simulink model "net"  (R2018b)
settings: Solver=VariableStepAuto  StartTime=0.0  StopTime=10.0  RelTol=1e-3
libraries: neural x107
(part 3 of 3)

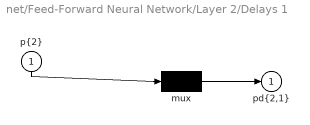
== system net/Feed-Forward Neural Network/Layer 2/Delays 1 ==
  "p{2}" : Inport  PortDimensions=100
      mask Display: e = 0.06;c1 = [120 230 180]/255;c2 = ([120 230 180]+0)/(256+128);c3 = ([120 230 180]+128)/(256+128);patch([0 1 1 0],[0 0 1 1],c1);patch([0 1 1 1-e 1-e 0+e],[0 0 1 1-e 0+e 0+e],c2);patch([0 0 1 1-e 0+e 0+e],[0 1 1 1-e 1-e 0+e],c3);plot([0 1 1 0 0],[0 0 1 1 0]);
  mux : Mux  Inputs=1
      mask Display: e = 0.06;c1 = [120 150 230]/255;c2 = ([120 150 230]+0)/383;c3 = ([120 150 230]+128)/383;patch([0 1 1 0],[0 0 1 1],c1);patch([0 1 1 1-e 1-e 0+e],[0 0 1 1-e 0+e 0+e],c2);patch([0 0 1 1-e 0+e 0+e],[0 1 1 1-e 1-e 0+e],c3);plot([0 1 1 0 0],[0 0 1 1 0]);disp('Mux')
  "pd{2,1}" : Outport
      mask Display: e = 0.06;c1 = [120 230 180]/255;c2 = ([120 230 180]+0)/(256+128);c3 = ([120 230 180]+128)/(256+128);patch([0 1 1 0],[0 0 1 1],c1);patch([0 1 1 1-e 1-e 0+e],[0 0 1 1-e 0+e 0+e],c2);patch([0 0 1 1-e 0+e 0+e],[0 1 1 1-e 1-e 0+e],c3);plot([0 1 1 0 0],[0 0 1 1 0]);
  wires:
  "p{2}"/1 -> mux/1
  mux/1 -> "pd{2,1}"/1

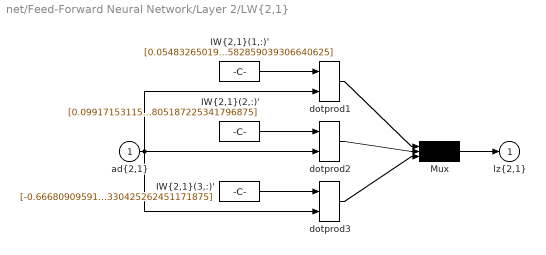
== system net/Feed-Forward Neural Network/Layer 2/LW{2,1} ==
  "ad{2,1}" : Inport  PortDimensions=100
      mask Display: e = 0.06;c1 = [120 230 180]/255;c2 = ([120 230 180]+0)/(256+128);c3 = ([120 230 180]+128)/(256+128);patch([0 1 1 0],[0 0 1 1],c1);patch([0 1 1 1-e 1-e 0+e],[0 0 1 1-e 0+e 0+e],c2);patch([0 0 1 1-e 0+e 0+e],[0 1 1 1-e 1-e 0+e],c3);plot([0 1 1 0 0],[0 0 1 1 0]);
  "IW{2,1}(1,:)'" : Constant  Value=[0.05483265019462690847973362906486727297306060791015625;0.012125815427491970499573881170363165438175201416015625;-0.1686587326797104047226838474671239964663982391357421875;-0.0202168258309454972054819421600768691860139369964599609375;0.09121870288483206745677733806587639264762401580810546875;0.353670820827776122285968085634522140026092529296875;-0.2475021717375649188408459622223745100200176239013671875;0.55673530010910587950689887293265201151371002197265625;0.015636698910315660615566457636305131018161773681640625;-0.0001195455807457557195760955437435768544673919677734375;0.3032284377369445227401456577354110777378082275390625;0.1307921379857321098061362363296211697161197662353515625;-0.244052362784950183094423437069053761661052703857421875;-0.6049096829452167423113451150129549205303192138671875;-0.3976379994996428468567728486959822475910186767578125;0.012026652977590514270733734747409471310675144195556640625;0.269113235915282855703622999499202705919742584228515625;-0.250837025003143809787076179418363608419895172119140625;0.379561693505631569944824832418817095458507537841796875;0.460939830487912372003478367332718335092067718505859375;-0.03214451578485445770727579883896396495401859283447265625;-0.0025710394266931051177049738498681108467280864715576171875;-0.52049228827995885904300621405127458274364471435546875;-0.09811246288179158170361660040725837461650371551513671875;-0.21610186479028847816863390107755549252033233642578125;0.0053971563130207067526811215429916046559810638427734375;-0.41390321109532390853047445489210076630115509033203125;-0.1428236061893602137917724803628516383469104766845703125;0.10957887134342043922163867364361067302525043487548828125;0.41999333485903267426664342565345577895641326904296875;0.11458371072683019853410968380558188073337078094482421875;0.1827573994210988372888238018276751972734928131103515625;-0.49626748851689661545805165587808005511760711669921875;-0.11629521544934078025601564831958967261016368865966796875;-0.0910286946376959449356291997901280410587787628173828125;0.323282162200989653388916167386923916637897491455078125;0.1194266060861080280819379595413920469582080841064453125;0.022955875877818811281461108819712535478174686431884765625;-0.0802221869070025850323446547918138094246387481689453125;0.000706058329053530810137662143688430660404264926910400390625;0.1055642718582814054695262484528939239680767059326171875;-0.11118762630784939648975750969839282333850860595703125;-0.288644173794616654138422973119304515421390533447265625;-0.04630920869394038186239725973791792057454586029052734375;-0.1142913256135923705247847692589857615530490875244140625;-0.203047329572125734298282395684509538114070892333984375;0.0981275451407927767899508353366400115191936492919921875;0.260774493761088965726457900018431246280670166015625;0.173697957117053325415412246002233587205410003662109375;-0.07354696279591499408212484922842122614383697509765625;0.01440227730156946883699475847606663592159748077392578125;0.02487745853650757954511618663673289120197296142578125;-0.12068044702138568113891636812695651315152645111083984375;-0.04503935934190887724337670761087792925536632537841796875;-0.03564348677737128046061343411565758287906646728515625;0.1220437472099527853597322746281861327588558197021484375;-0.12375763757898268491164373017454636283218860626220703125;0.08675788736643898213518610873506986536085605621337890625;0.006363833838641287654613876156872720457613468170166015625;0.063090967375005579942381928049144335091114044189453125;-0.1555091428616292292819167641937383450567722320556640625;0.2683263482211171169211638698470778763294219970703125;-0.157252983216918773567982725580804981291294097900390625;0.0257458496007904429070389795697337831370532512664794921875;-0.0788007832297293597800802444908185862004756927490234375;-0.252624347104402013908241997341974638402462005615234375;0.054402396917277169585691609654531930573284626007080078125;-0.0047298987202938069795976616660482250154018402099609375 ...(+1842 chars)]
      mask Display: e = 0.06;c1 = [120 150 230]/255;c2 = ([120 150 230]+0)/383;c3 = ([120 150 230]+128)/383;patch([0 1 1 0],[0 0 1 1],c1);patch([0 1 1 1-e 1-e 0+e],[0 0 1 1-e 0+e 0+e],c2);patch([0 0 1 1-e 0+e 0+e],[0 1 1 1-e 1-e 0+e],c3);plot([0 1 1 0 0],[0 0 1 1 0]);disp('weights');
  "IW{2,1}(2,:)'" : Constant  Value=[0.099171531150535674470347657916136085987091064453125;1.2131689394934774828271883961861021816730499267578125;-0.37240338475430057041393183681066147983074188232421875;-0.094913748072395331956130348771694116294384002685546875;0.051589458935953298734933269997782190330326557159423828125;-0.24520420939644782531985356399673037230968475341796875;-0.1055938873189418980569342920716735534369945526123046875;0.477008291154038366332912346479133702814579010009765625;-0.454310030393080932498151014442555606365203857421875;-0.0911311052745233662886192860241862945258617401123046875;-0.1904046234671627757517597956393728964030742645263671875;-0.25870834412288445935956815446843393146991729736328125;-0.149542546544342791481341237158630974590778350830078125;-0.8359853157817933588802361555281095206737518310546875;0.32953841214769286072083787075825966894626617431640625;-0.06085508872867458063371515208928030915558338165283203125;0.191876391730093853738026155042462050914764404296875;-0.2481052420968397342893041468414594419300556182861328125;-0.0065443612925791504186801006426321691833436489105224609375;-0.00809415123531025994252363631176194758154451847076416015625;-0.09419575984834784032617704951917403377592563629150390625;0.221952180974647250710773960236110724508762359619140625;0.022914457430139034688210131207597441971302032470703125;0.02997399214734901284895585149570251815021038055419921875;0.00428522437911511670793895945053009199909865856170654296875;0.331100008904916476293323057689121924340724945068359375;-1.4668779706923655847816689856699667870998382568359375;-0.127276279824535765161641620579757727682590484619140625;-0.08159542052484136664958214169018901884555816650390625;0.77968582590737744997255731504992581903934478759765625;0.039800757264523693723656805332211661152541637420654296875;-0.124745319562124479251252751055289991199970245361328125;-0.168120744341439476432498167923768050968647003173828125;-0.2863807394242738890710597843280993402004241943359375;-0.0984388388261607516493967295900802128016948699951171875;-0.09328726024501508840014452061950578354299068450927734375;0.0467612750197999582635333126745535992085933685302734375;-0.093564077709736570565013380473828874528408050537109375;-0.228966853567604766706011787391616962850093841552734375;0.0078419474229698242495611992808335344307124614715576171875;-0.14171721139573112413501121409353800117969512939453125;-0.259579624037585887652568317207624204456806182861328125;-0.1149621114330283688786948914639651775360107421875;-0.08159460516733203772066218562031281180679798126220703125;0.283378362874139977378717958345077931880950927734375;-0.1983318672905276247586670024247723631560802459716796875;0.0140898281504987545054152775492184446193277835845947265625;0.37684717730570771454523537613567896187305450439453125;0.22095677284512416083117614107322879135608673095703125;-0.0784169028023156966522577704381546936929225921630859375;-0.2072775950195665795039445811198675073683261871337890625;-0.1636375183813505718166680935610202141106128692626953125;-0.0867452439461409152698934121872298419475555419921875;-0.1875034659212668486372166398723493330180644989013671875;0.14231978925192689811041191205731593072414398193359375;0.10864480738682284755025619915613788180053234100341796875;-0.30765227903146630250574844467337243258953094482421875;0.02874007293482323810440703937274520285427570343017578125;0.08352802605819960313215943870090995915234088897705078125;0.1680991649529957887576614439240074716508388519287109375;0.01398647729947304074737957080287742428481578826904296875;-0.0370100993996946014963356219595880247652530670166015625;0.10127254256547468802551748012774623930454254150390625;-0.481585676713659649461618528221151791512966156005859375;-0.1687844003476044463241123594343662261962890625;-0.40014042229849733356417118557146750390529632568359375;0.06211113427337373871228720645376597531139850616455078125;-0.1038134994151001244677701151886139996349811553955078125;0.213983363620779354352663403915357775986194610595703125 ...(+1798 chars)]
      mask Display: e = 0.06;c1 = [120 150 230]/255;c2 = ([120 150 230]+0)/383;c3 = ([120 150 230]+128)/383;patch([0 1 1 0],[0 0 1 1],c1);patch([0 1 1 1-e 1-e 0+e],[0 0 1 1-e 0+e 0+e],c2);patch([0 0 1 1-e 0+e 0+e],[0 1 1 1-e 1-e 0+e],c3);plot([0 1 1 0 0],[0 0 1 1 0]);disp('weights');
  "IW{2,1}(3,:)'" : Constant  Value=[-0.6668090959146180107808277170988731086254119873046875;-2.4810549698668413753921413444913923740386962890625;0.356625395162307678997848370272549800574779510498046875;0.55467576706450116841295994163374416530132293701171875;0.376624318268824309630105062751681543886661529541015625;-0.18656430021685499465178281752741895616054534912109375;0.50895678970246549521760925927083007991313934326171875;-1.4842829602800653443495093597448430955410003662109375;-0.240248190371791403574519563335343264043331146240234375;-0.444989753763534279240587920867255888879299163818359375;0.0218716064216709464573806798171062837354838848114013671875;-0.0497289414621266967486690191435627639293670654296875;-0.0680342482120100122688910460055922158062458038330078125;1.732232709587925523209150924230925738811492919921875;-2.235752551283036293483519330038689076900482177734375;0.1491891902804252101333304381114430725574493408203125;1.08044913398688446903861404280178248882293701171875;0.74215459449798670821252244422794319689273834228515625;1.0798558137761562480960719767608679831027984619140625;0.37414551441459631409003350199782289564609527587890625;-0.0250704934851594153644160911653671064414083957672119140625;-0.142905062667793736341792509847437031567096710205078125;-0.27744812179227384962842961613205261528491973876953125;-0.228452759547958683672419510912732221186161041259765625;0.1257390488800839978278389708066242747008800506591796875;-0.71113576801938138682857015737681649625301361083984375;-3.17429107110410146930234986939467489719390869140625;0.223439776571520198888975983209093101322650909423828125;-0.1609900880566176029073943709590821526944637298583984375;-1.548756567594530064724267504061572253704071044921875;-0.045447650509174597477368706677225418388843536376953125;-0.176225662826850870690265082885161973536014556884765625;0.4931829358689612252675260606338270008563995361328125;0.94899716212398488313084499168326146900653839111328125;0.491499846390909655990952842330443672835826873779296875;0.6302359044320107184233847874565981328487396240234375;-0.360333300085248720012742751350742764770984649658203125;0.1485194621129110881252444187339278869330883026123046875;-0.4857472873466124330121829189010895788669586181640625;-0.198753972132814038520365329532069154083728790283203125;-0.40906488863752621387703811706160195171833038330078125;0.0640141232475315014038841354704345576465129852294921875;0.37617694526365019758173957598046399652957916259765625;0.1611495237603486063715507725646602921187877655029296875;1.5589853397094615150564322902937419712543487548828125;0.41126513980483092591811100646737031638622283935546875;-0.59003217775567773362155321592581458389759063720703125;-0.431868284626862497521671002687071450054645538330078125;-0.420966915679006958850294495277921669185161590576171875;1.035587686603992807476970483548939228057861328125;-0.47756041669068360899785830042674206197261810302734375;0.014826678348172021848494495088743860833346843719482421875;0.127697651030679482087037968085496686398983001708984375;-0.118164754644348446444013234213343821465969085693359375;0.712820834475847764366562842042185366153717041015625;-0.331796330984266918395775292083271779119968414306640625;1.13275741351497316600216436199843883514404296875;0.4295925267533469149583424950833432376384735107421875;0.091423864512593044917565521245705895125865936279296875;0.2318091536341502223450561359641142189502716064453125;0.537202432265116325282860998413525521755218505859375;-0.19903371433536809487208074642694555222988128662109375;-0.48114181483564910646322232423699460923671722412109375;1.268583711686357862191698586684651672840118408203125;-0.396701194118952271683298249627114273607730865478515625;0.37798994191761747796221015960327349603176116943359375;-0.612809070489451102048406028188765048980712890625;-0.46642957625478798089346810229471884667873382568359375;-0.165155559902059045906952405857737176120281219482421875;0.810593550098296145023368808324448764324188232421875 ...(+1676 chars)]
      mask Display: e = 0.06;c1 = [120 150 230]/255;c2 = ([120 150 230]+0)/383;c3 = ([120 150 230]+128)/383;patch([0 1 1 0],[0 0 1 1],c1);patch([0 1 1 1-e 1-e 0+e],[0 0 1 1-e 0+e 0+e],c2);patch([0 0 1 1-e 0+e 0+e],[0 1 1 1-e 1-e 0+e],c3);plot([0 1 1 0 0],[0 0 1 1 0]);disp('weights');
  Mux : Mux  Inputs=3
      mask Display: e = 0.06;c1 = [120 150 230]/255;c2 = ([120 150 230]+0)/383;c3 = ([120 150 230]+128)/383;patch([0 1 1 0],[0 0 1 1],c1);patch([0 1 1 1-e 1-e 0+e],[0 0 1 1-e 0+e 0+e],c2);patch([0 0 1 1-e 0+e 0+e],[0 1 1 1-e 1-e 0+e],c3);plot([0 1 1 0 0],[0 0 1 1 0]);disp('Mux');
  dotprod1 : neural/Weight Functions/dotprod
  dotprod2 : neural/Weight Functions/dotprod
  dotprod3 : neural/Weight Functions/dotprod
  "lz{2,1}" : Outport
      mask Display: e = 0.06;c1 = [120 230 180]/255;c2 = ([120 230 180]+0)/(256+128);c3 = ([120 230 180]+128)/(256+128);patch([0 1 1 0],[0 0 1 1],c1);patch([0 1 1 1-e 1-e 0+e],[0 0 1 1-e 0+e 0+e],c2);patch([0 0 1 1-e 0+e 0+e],[0 1 1 1-e 1-e 0+e],c3);plot([0 1 1 0 0],[0 0 1 1 0]);
  wires:
  "IW{2,1}(1,:)'"/1 -> dotprod1/1
  "ad{2,1}"/1 -> dotprod1/2, dotprod2/2, dotprod3/2
  dotprod1/1 -> Mux/1
  "IW{2,1}(2,:)'"/1 -> dotprod2/1
  dotprod2/1 -> Mux/2
  "IW{2,1}(3,:)'"/1 -> dotprod3/1
  dotprod3/1 -> Mux/3
  Mux/1 -> "lz{2,1}"/1
